simulink library "BCM"  (R2021a)
settings: Solver=VariableStepAuto  StartTime=0.0  StopTime=10.0  RelTol=1e-3
libraries: simulink x2, $bdroot x1
settings Model: Creator=Sai229  LastModifiedBy=Sai229

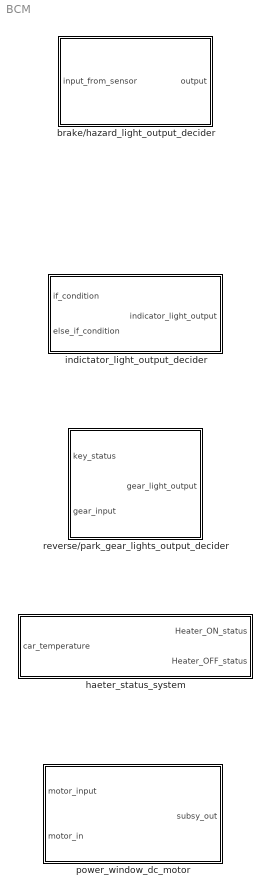
== system BCM ==
  brake/hazard_light_output_decider : Subsystem  mask(Brake and Hazard Light Output decider){}
      mask help: This system decides the output of brake and hazard lights, whether they are on or off. Connect the brake sensor or the hazard switch sensor to the input and based on the input the output port will turn on or turn off brake lights or hazard lights
  haeter_status_system : Subsystem
  indictator_light_output_decider : Subsystem  mask(Indicator lights output decider){}
      mask help: This system decides the output of indicator lights (left and right indicators) whether they are on or off. Connect the signal to if_condition input when you want the indicator lights to blink. Connect the signal to else_if_condition input when you want the indicator lights to remain in off condition. The output of this system can be connected to merge blocks.
  power_window_dc_motor : Subsystem
  reverse/park_gear_lights_output_decider : Subsystem  mask(Reverse/Park gear lights output decider){gear_option=Neutral}
      mask prompts: gear_option "Enter the gear option"
      mask help: This system decides the output of the reverse gear lights and park gear lights. Connect the key status to key_input and gear sensor input to gear_option button. Connect the output to the gear lights
      mask TypeOptions gear_option: Neutral | Drive | Park | Reverse

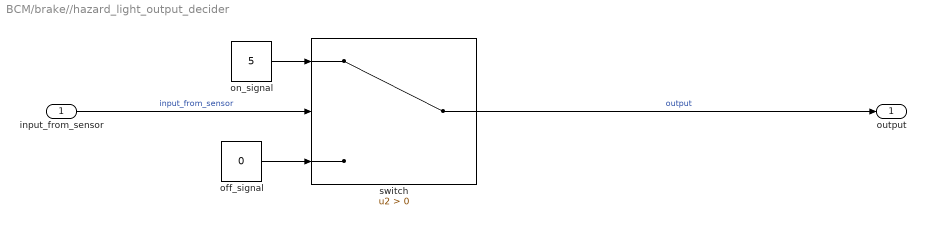
== system BCM/brake//hazard_light_output_decider ==
  input_from_sensor : Inport
  off_signal : Constant  Value=0  VectorParams1D=off  SampleTime=-1
  on_signal : Constant  Value=5  VectorParams1D=off  SampleTime=-1
  switch : Switch  Criteria=u2 > Threshold
  output : Outport
  wires:
  on_signal/1 -> switch/1
  off_signal/1 -> switch/3
  switch/1 -> output/1  "output"
  input_from_sensor/1 -> switch/2  "input_from_sensor"

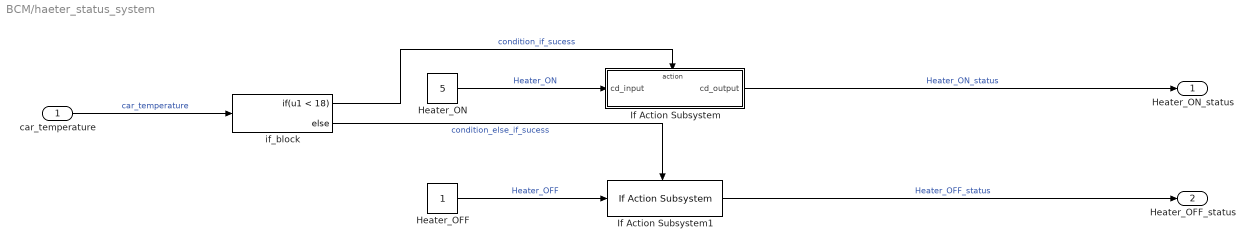
== system BCM/haeter_status_system ==
  car_temperature : Inport
  Heater_OFF : Constant
  Heater_ON : Constant  Value=5
  If Action Subsystem : Subsystem  TreatAsAtomicUnit=on
  If Action Subsystem1 : $bdroot/haeter_status_system/If Action Subsystem  SystemSampleTime=-1  VariantActivationTime=update diagram  Latency=0  AutoFrameSizeCalculation=off
  if_block : If  IfExpression=u1 < 18
  Heater_ON_status : Outport
  Heater_OFF_status : Outport  Port=2
  wires:
  Heater_OFF/1 -> If Action Subsystem1/1  "Heater_OFF"
  car_temperature/1 -> if_block/1  "car_temperature"
  If Action Subsystem/1(cd_output) -> Heater_ON_status/1  "Heater_ON_status"
  if_block/2 -> If Action Subsystem1/Action  "condition_else_if_sucess"
  Heater_ON/1 -> If Action Subsystem/1(cd_input)  "Heater_ON"
  If Action Subsystem1/1 -> Heater_OFF_status/1  "Heater_OFF_status"
  if_block/1 -> If Action Subsystem/Action  "condition_if_sucess"

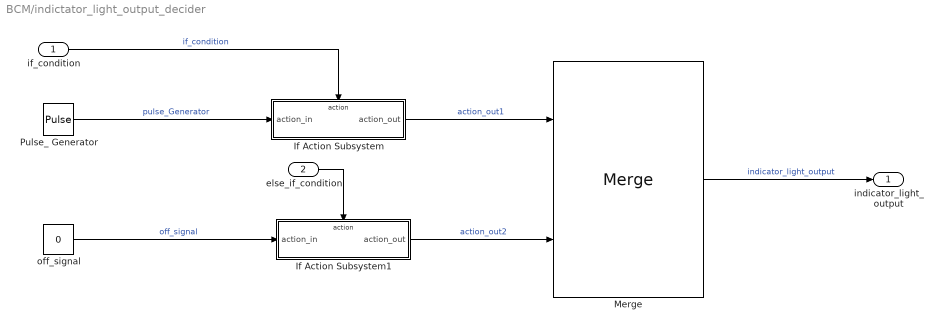
== system BCM/indictator_light_output_decider ==
  if_condition : Inport
  else_if_condition : Inport  Port=2
  If Action Subsystem : Subsystem  TreatAsAtomicUnit=on
  If Action Subsystem1 : Subsystem  TreatAsAtomicUnit=on
  Merge : Merge
  Pulse_ Generator : DiscretePulseGenerator  PulseType=Time based  Amplitude=5  Period=0.1  PulseWidth=50
  off_signal : Constant  Value=0
  indicator_light_output : Outport
  wires:
  else_if_condition/1 -> If Action Subsystem1/Action
  Pulse_ Generator/1 -> If Action Subsystem/1(action_in)  "pulse_Generator"
  off_signal/1 -> If Action Subsystem1/1(action_in)  "off_signal"
  if_condition/1 -> If Action Subsystem/Action  "if_condition"
  If Action Subsystem/1(action_out) -> Merge/1  "action_out1"
  If Action Subsystem1/1(action_out) -> Merge/2  "action_out2"
  Merge/1 -> indicator_light_output/1  "indicator_light_output"

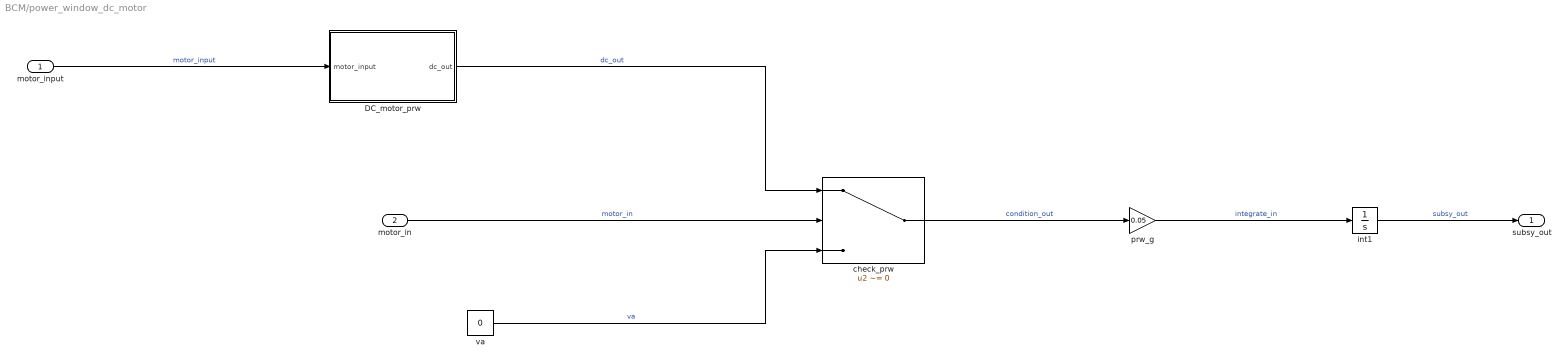
== system BCM/power_window_dc_motor ==
  motor_input : Inport
  motor_in : Inport  Port=2
  DC_motor_prw : Subsystem
  check_prw : Switch  Criteria=u2 ~= 0
  int1 : Integrator  InitialCondition=0.0001
      settings: AttributesFormatString=%<InitialCondition>
  prw_g : Gain  Gain=0.05
  va : Constant  Value=0
  subsy_out : Outport
  wires:
  prw_g/1 -> int1/1  "integrate_in"
  check_prw/1 -> prw_g/1  "condition_out"
  va/1 -> check_prw/3  "va"
  DC_motor_prw/1(dc_out) -> check_prw/1  "dc_out"
  motor_input/1 -> DC_motor_prw/1(motor_input)  "motor_input"
  int1/1 -> subsy_out/1  "subsy_out"
  motor_in/1 -> check_prw/2  "motor_in"

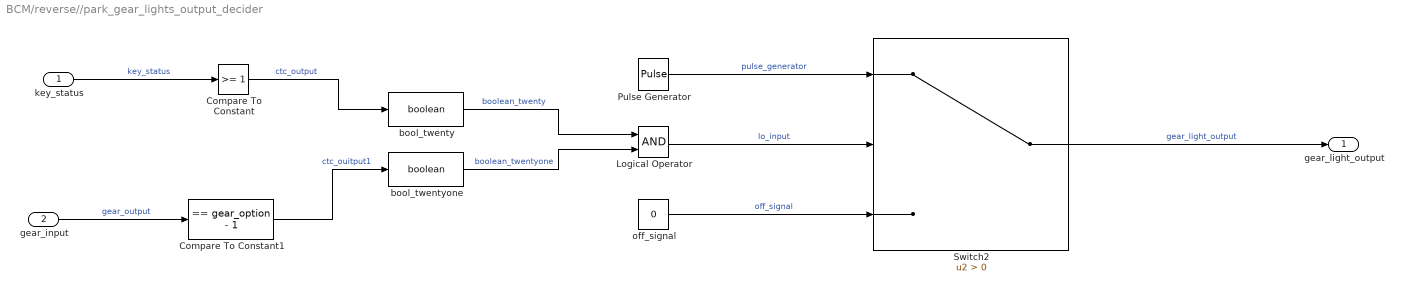
== system BCM/reverse//park_gear_lights_output_decider ==
  key_status : Inport
  gear_input : Inport  Port=2
  Compare To Constant : simulink/Logic and Bit Operations/Compare To Constant  relop=>=  const=1  OutDataTypeStr=boolean
  Compare To Constant1 : simulink/Logic and Bit Operations/Compare To Constant  relop===  const=gear_option - 1  OutDataTypeStr=boolean
  Logical Operator : Logic  AllPortsSameDT=off  OutDataTypeStr=boolean
  Pulse Generator : DiscretePulseGenerator  PulseType=Time based  Amplitude=5  Period=0.1  PulseWidth=50
  Switch2 : Switch  Criteria=u2 > Threshold
  bool_twenty : DataTypeConversion  OutDataTypeStr=boolean
  bool_twentyone : DataTypeConversion  OutDataTypeStr=boolean
  off_signal : Constant  Value=0
  gear_light_output : Outport
  wires:
  Compare To Constant1/1 -> bool_twentyone/1  "ctc_ouitput1"
  off_signal/1 -> Switch2/3  "off_signal"
  Pulse Generator/1 -> Switch2/1  "pulse_generator"
  gear_input/1 -> Compare To Constant1/1  "gear_output"
  key_status/1 -> Compare To Constant/1  "key_status"
  Switch2/1 -> gear_light_output/1  "gear_light_output"
  Logical Operator/1 -> Switch2/2  "lo_input"
  Compare To Constant/1 -> bool_twenty/1  "ctc_output"
  bool_twenty/1 -> Logical Operator/1  "boolean_twenty"
  bool_twentyone/1 -> Logical Operator/2  "boolean_twentyone"

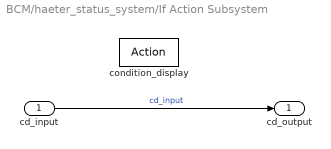
== system BCM/haeter_status_system/If Action Subsystem ==
  cd_input : Inport
  condition_display : ActionPort  ActionPortLabel=if(u1 < 18)
  cd_output : Outport
  wires:
  cd_input/1 -> cd_output/1  "cd_input"

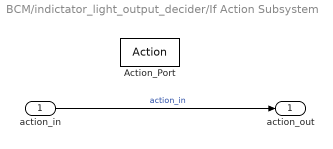
== system BCM/indictator_light_output_decider/If Action Subsystem ==
  action_in : Inport
  Action_Port : ActionPort
  action_out : Outport
  wires:
  action_in/1 -> action_out/1  "action_in"

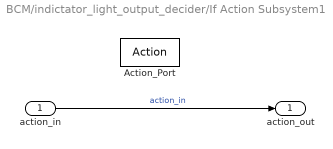
== system BCM/indictator_light_output_decider/If Action Subsystem1 ==
  action_in : Inport
  Action_Port : ActionPort
  action_out : Outport
  wires:
  action_in/1 -> action_out/1  "action_in"

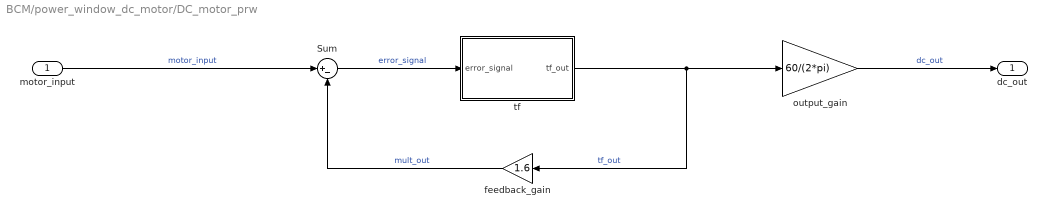
== system BCM/power_window_dc_motor/DC_motor_prw ==
  motor_input : Inport
  Sum : Sum  Inputs=|+-
  feedback_gain : Gain  Gain=1.6
  output_gain : Gain  Gain=60/(2*pi)
  tf : Subsystem  TreatAsAtomicUnit=on  mask{TL=20}
      mask prompts: TL "Enter value of TL"
      mask Display: disp("Transfer subsystem");
  dc_out : Outport
  wires:
  output_gain/1 -> dc_out/1  "dc_out"
  feedback_gain/1 -> Sum/2  "mult_out"
  tf/1(tf_out) -> output_gain/1, feedback_gain/1  "tf_out"
  Sum/1 -> tf/1(error_signal)  "error_signal"
  motor_input/1 -> Sum/1  "motor_input"

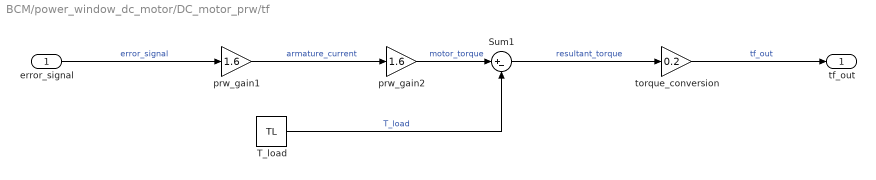
== system BCM/power_window_dc_motor/DC_motor_prw/tf ==
  error_signal : Inport
  Sum1 : Sum  Inputs=|+-
  T_load : Constant  Value=TL
  prw_gain1 : Gain  Gain=1.6
  prw_gain2 : Gain  Gain=1.6
  torque_conversion : Gain  Gain=0.2
  tf_out : Outport
  wires:
  torque_conversion/1 -> tf_out/1  "tf_out"
  prw_gain2/1 -> Sum1/1  "motor_torque"
  error_signal/1 -> prw_gain1/1  "error_signal"
  T_load/1 -> Sum1/2  "T_load"
  prw_gain1/1 -> prw_gain2/1  "armature_current"
  Sum1/1 -> torque_conversion/1  "resultant_torque"
